simulink model "observerModel_GVS_MS"  (R2023b)
settings: Solver=ode15s  StartTime=0.0  StopTime=duration  MaxStep=0.02  RelTol=0.02  AbsTol=0.02  EnableMultiTasking=on
values from neighbouring files (symbols this model uses):
  beta1 = s(8)    [Observer_Analysis.m]
  beta2 = s(7)    [Observer_Analysis.m]
  delta_t = time(2) - time (1)    [Observer_Analysis.m]
  df = 1    [Observer_Analysis.m]
  f_oto = 2    [Observer_Analysis.m]
  f_scc = 2    [Observer_Analysis.m]
  f_visO = 0.2    [Observer_Analysis.m]
  f_visV = 2    [Observer_Analysis.m]
  f_visX = 2    [Observer_Analysis.m]
  GG0 = [0 0 -hypo]'    [Observer_Analysis.m]
  IrregDepol = tf(num,den)    [Observer_Analysis.m]
  IrregHyperpol = tf(num,den)    [Observer_Analysis.m]
  IrregSCC2Physical = inv(IrregSCCnf)    [Observer_Analysis.m]
  kaa = -3.2*[1 1 1]'    [Observer_Analysis.m]
  Kea = s(1)^(1/2)*[1 1 1]    [Observer_Analysis.m]
  Kef = s(3)^(1/2)*[1 1 1]    [Observer_Analysis.m]
  Kew = s(2)^(1/2)*[1 1 1]    [Observer_Analysis.m]
  Kfast = s(4)    [Observer_Analysis.m]
  kfg = 4*[1 1 1]'    [Observer_Analysis.m]
  kfw = 8*[1 1 1]'    [Observer_Analysis.m]
  kgvg = 5*[1 1 1]'    [Observer_Analysis.m]
  KLeft = 1-KRight    (= 0.5)    [Observer_Analysis.m]
  KReg = s2(2)    [Observer_Analysis.m]
  KRight = 0.5    [Observer_Analysis.m]
  KS = s2(1)*pi/180    [Observer_Analysis.m]
  kwg = 1*[1 1 1]'    [Observer_Analysis.m]
  kwvw = 10*[1 1 1]'    [Observer_Analysis.m]
  kww = 2.28*[1 1 1]'    [Observer_Analysis.m]
  kxdotva = 0.75*[1 1 1]'    [Observer_Analysis.m]
  kxvv = 0.1*[1 1 1]'    [Observer_Analysis.m]
  LeftSide_CurrentMult = s2(4)    [Observer_Analysis.m]
  ms_exp = s(6)    [Observer_Analysis.m]
  oto_a = 60*[1 1 1]'    [Observer_Analysis.m]
  oto_Ka = 1.3*[1 1 1]'    [Observer_Analysis.m]
  Q0 = [cos(E_angle/2) E(1)*sin(E_angle/2) E(2)*sin(E_angle/2) E(3)*sin(E_angle/2)]'    [Observer_Analysis.m]
  RegDepol = tf(num,den)    [Observer_Analysis.m]
  RegHyperpol = tf(num,den)    [Observer_Analysis.m]
  RegSCC2Physical = inv(RegSCCnf)    [Observer_Analysis.m]
  tau_a = tau_a_value*[1 1 1]'    [Observer_Analysis.m]
  tau_scc = tau_scc_value*[1 1 1]'    [Observer_Analysis.m]
  x_leak = 0.6    [Observer_Analysis.m]
  y_leak = 0.6    [Observer_Analysis.m]
  z_leak = 10    [Observer_Analysis.m]
(part 3 of 3)

== system observerModel_GVS_MS/Subsystem5/Subsystem4/Matrix Multiplication ==
  D_Cos : Inport
  a_esr_head : Inport  Port=2
  Demux : Demux  Outputs=3
      settings: DisplayOption=none
  Math Function : Math  Operator=transpose  SignedPower=on
  Mux : Mux  Inputs=3
  Product : Product  Multiplication=Matrix(*)  RndMeth=Zero
  a_est_world : Outport
  wires:
  Product/1 -> Demux/1
  Demux/1 -> Mux/1
  Demux/2 -> Mux/2
  Demux/3 -> Mux/3
  D_Cos/1 -> Math Function/1
  Mux/1 -> a_est_world/1
  a_esr_head/1 -> Product/2
  Math Function/1 -> Product/1

== system observerModel_GVS_MS/To VR (actual)/Limbic to VR Displacement/Transform Axes Translation ==
  head_cord : Inport
  Demux2 : Demux  Outputs=3
  Mux2 : Mux  Inputs=3
  VR_cord : Outport
  wires:
  Demux2/1 -> Mux2/3
  Demux2/2 -> Mux2/1
  Demux2/3 -> Mux2/2
  head_cord/1 -> Demux2/1
  Mux2/1 -> VR_cord/1

== system observerModel_GVS_MS/To VR (est)/Limbic to VR Estimated Displacement/Transform Axes Translation Est ==
  head_cord : Inport
  Demux2 : Demux  Outputs=3
  Mux2 : Mux  Inputs=3
  VR_cord : Outport
  wires:
  Demux2/1 -> Mux2/3
  Demux2/2 -> Mux2/1
  Demux2/3 -> Mux2/2
  head_cord/1 -> Demux2/1
  Mux2/1 -> VR_cord/1

== system observerModel_GVS_MS/Quaternion Rotator/Head to Limbic Angular Velocity Transform/Quaternion Integrator1/delta_q ==
  omega : Inport
  q : Inport  Port=2
  C : Subsystem
  Constant : Constant  Value=delta_t
  K : Subsystem
  Product : Product  RndMeth=Zero
  Product1 : Product  RndMeth=Zero
  Product2 : Product  RndMeth=Zero
  Sum : Sum
  Z : Subsystem
  delta_q : Outport
  wires:
  q/1 -> C/2(q), Z/1(q), Product1/1
  Z/1(z) -> Product/1
  Product/1 -> Product1/2
  Product1/1 -> Sum/2
  C/1(C) -> Sum/1
  Sum/1 -> Product2/2
  Constant/1 -> Product2/1
  omega/1 -> C/1(omega)
  Product2/1 -> delta_q/1
  K/1(K) -> Product/2

== system observerModel_GVS_MS/Quaternion Rotator/Head to Limbic Angular Velocity Transform/Quaternion to Direction Cosine1/A1 ==
  q : Inport
  Demux : Demux
  Gain : Gain  Gain=2
  Product : Product  RndMeth=Zero
  Product1 : Product  RndMeth=Zero
  Sum : Sum  Inputs=+-
  A21 : Outport
  wires:
  q/1 -> Demux/1
  Sum/1 -> Gain/1
  Gain/1 -> A21/1
  Product/1 -> Sum/1
  Product1/1 -> Sum/2
  Demux/2 -> Product/1
  Demux/3 -> Product/2
  Demux/1 -> Product1/1
  Demux/4 -> Product1/2

== system observerModel_GVS_MS/Quaternion Rotator/Head to Limbic Angular Velocity Transform/Quaternion to Direction Cosine1/A11 ==
  q : Inport
  Demux : Demux
  Product{,1..3} (4 alike) : Product  RndMeth=Zero
  Sum : Sum  Inputs=++--
  A11 : Outport
  wires:
  Demux/1 -> Product/1, Product/2
  Demux/2 -> Product1/1, Product1/2
  Demux/3 -> Product2/1, Product2/2
  Demux/4 -> Product3/1, Product3/2
  Product/1 -> Sum/1
  Product1/1 -> Sum/2
  Product2/1 -> Sum/3
  Product3/1 -> Sum/4
  q/1 -> Demux/1
  Sum/1 -> A11/1

== system observerModel_GVS_MS/Quaternion Rotator/Head to Limbic Angular Velocity Transform/Quaternion to Direction Cosine1/A12 ==
  q : Inport
  Demux : Demux
  Gain : Gain  Gain=2
  Product : Product  RndMeth=Zero
  Product1 : Product  RndMeth=Zero
  Sum : Sum
  A12 : Outport
  wires:
  q/1 -> Demux/1
  Sum/1 -> Gain/1
  Gain/1 -> A12/1
  Demux/2 -> Product/1
  Demux/3 -> Product/2
  Demux/1 -> Product1/1
  Demux/4 -> Product1/2
  Product/1 -> Sum/1
  Product1/1 -> Sum/2

== system observerModel_GVS_MS/Quaternion Rotator/Head to Limbic Angular Velocity Transform/Quaternion to Direction Cosine1/A13 ==
  q : Inport
  Demux : Demux
  Gain : Gain  Gain=2
  Product : Product  RndMeth=Zero
  Product1 : Product  RndMeth=Zero
  Sum : Sum  Inputs=+-
  A13 : Outport
  wires:
  q/1 -> Demux/1
  Sum/1 -> Gain/1
  Gain/1 -> A13/1
  Product/1 -> Sum/1
  Product1/1 -> Sum/2
  Demux/2 -> Product/1
  Demux/4 -> Product/2
  Demux/1 -> Product1/1
  Demux/3 -> Product1/2

== system observerModel_GVS_MS/Quaternion Rotator/Head to Limbic Angular Velocity Transform/Quaternion to Direction Cosine1/A22 ==
  q : Inport
  Demux : Demux
  Product{,1..3} (4 alike) : Product  RndMeth=Zero
  Sum : Sum  Inputs=+-+-
  A22 : Outport
  wires:
  Demux/1 -> Product/1, Product/2
  Demux/2 -> Product1/1, Product1/2
  Demux/3 -> Product2/1, Product2/2
  Demux/4 -> Product3/1, Product3/2
  Product/1 -> Sum/1
  Product1/1 -> Sum/2
  Product2/1 -> Sum/3
  Product3/1 -> Sum/4
  q/1 -> Demux/1
  Sum/1 -> A22/1

== system observerModel_GVS_MS/Quaternion Rotator/Head to Limbic Angular Velocity Transform/Quaternion to Direction Cosine1/A23 ==
  q : Inport
  Demux : Demux
  Gain : Gain  Gain=2
  Product : Product  RndMeth=Zero
  Product1 : Product  RndMeth=Zero
  Sum : Sum
  A23 : Outport
  wires:
  q/1 -> Demux/1
  Sum/1 -> Gain/1
  Gain/1 -> A23/1
  Product/1 -> Sum/1
  Product1/1 -> Sum/2
  Demux/3 -> Product1/1
  Demux/4 -> Product1/2
  Demux/1 -> Product/1
  Demux/2 -> Product/2

== system observerModel_GVS_MS/Quaternion Rotator/Head to Limbic Angular Velocity Transform/Quaternion to Direction Cosine1/A31 ==
  q : Inport
  Demux : Demux
  Gain : Gain  Gain=2
  Product : Product  RndMeth=Zero
  Product1 : Product  RndMeth=Zero
  Sum : Sum
  A31 : Outport
  wires:
  q/1 -> Demux/1
  Sum/1 -> Gain/1
  Gain/1 -> A31/1
  Product/1 -> Sum/1
  Product1/1 -> Sum/2
  Demux/1 -> Product/1
  Demux/3 -> Product/2
  Demux/2 -> Product1/1
  Demux/4 -> Product1/2

== system observerModel_GVS_MS/Quaternion Rotator/Head to Limbic Angular Velocity Transform/Quaternion to Direction Cosine1/A32 ==
  q : Inport
  Demux : Demux
  Gain : Gain  Gain=2
  Product : Product  RndMeth=Zero
  Product1 : Product  RndMeth=Zero
  Sum : Sum  Inputs=+-
  A32 : Outport
  wires:
  q/1 -> Demux/1
  Sum/1 -> Gain/1
  Gain/1 -> A32/1
  Product/1 -> Sum/1
  Product1/1 -> Sum/2
  Demux/3 -> Product/1
  Demux/4 -> Product/2
  Demux/1 -> Product1/1
  Demux/2 -> Product1/2

== system observerModel_GVS_MS/Quaternion Rotator/Head to Limbic Angular Velocity Transform/Quaternion to Direction Cosine1/A33 ==
  q : Inport
  Demux : Demux
  Product{,1..3} (4 alike) : Product  RndMeth=Zero
  Sum : Sum  Inputs=+--+
  A33 : Outport
  wires:
  Demux/1 -> Product/1, Product/2
  Demux/2 -> Product1/1, Product1/2
  Demux/3 -> Product2/1, Product2/2
  Demux/4 -> Product3/1, Product3/2
  Product/1 -> Sum/1
  Product1/1 -> Sum/2
  Product2/1 -> Sum/3
  Product3/1 -> Sum/4
  q/1 -> Demux/1
  Sum/1 -> A33/1

== system observerModel_GVS_MS/Quaternion Rotator/Quaternion Integrator/delta_q/C ==
  omega : Inport
  q : Inport  Port=2
  C1 : Subsystem
  C2 : Subsystem
  C3 : Subsystem
  C4 : Subsystem
  Mux : Mux
  C : Outport
  wires:
  omega/1 -> C1/1(omega), C2/1(omega), C3/1(omega), C4/1(omega)
  q/1 -> C4/2(q), C3/2(q), C2/2(q), C1/2(q)
  C1/1(c1) -> Mux/1
  C2/1(c2) -> Mux/2
  C3/1(c3) -> Mux/3
  C4/1(c4) -> Mux/4
  Mux/1 -> C/1

== system observerModel_GVS_MS/Quaternion Rotator/Quaternion Integrator/delta_q/K ==
  Product : Product  RndMeth=Zero
  k : Constant  Value=1/delta_t
  value : Constant  Value=0.9
  K : Outport
  wires:
  k/1 -> Product/1
  Product/1 -> K/1
  value/1 -> Product/2

== system observerModel_GVS_MS/Quaternion Rotator/Quaternion Integrator/delta_q/Z ==
  q : Inport
  Constant : Constant
  Demux : Demux
  Product{,1..3} (4 alike) : Product  RndMeth=Zero
  Sum : Sum  Inputs=++++
  Sum1 : Sum  Inputs=+-
  z : Outport
  wires:
  Demux/1 -> Product/1, Product/2
  Demux/2 -> Product1/1, Product1/2
  Demux/3 -> Product2/1, Product2/2
  Demux/4 -> Product3/1, Product3/2
  q/1 -> Demux/1
  Product/1 -> Sum/1
  Product1/1 -> Sum/2
  Product2/1 -> Sum/3
  Product3/1 -> Sum/4
  Sum/1 -> Sum1/2
  Constant/1 -> Sum1/1
  Sum1/1 -> z/1

== system observerModel_GVS_MS/Quaternion Rotator/Rotation/Azimuthal Integrator/Matrix Multiplication1 ==
  D_Cos : Inport
  omega_rad : Inport  Port=2
  Demux : Demux  Outputs=3
      settings: DisplayOption=none
  Mux : Mux  Inputs=3
  Product : Product  Multiplication=Matrix(*)  RndMeth=Zero
  omega_rad' : Outport
  wires:
  Product/1 -> Demux/1
  Demux/1 -> Mux/1
  Demux/2 -> Mux/2
  Demux/3 -> Mux/3
  D_Cos/1 -> Product/1
  Mux/1 -> omega_rad'/1
  omega_rad/1 -> Product/2

== system observerModel_GVS_MS/Quaternion Rotator2/Head to Limbic Angular Velocity Transform Rotation Matrix/Quaternion Integrator1/delta_q ==
  omega : Inport
  q : Inport  Port=2
  C : Subsystem
  Constant : Constant  Value=delta_t
  K : Subsystem
  Product : Product  RndMeth=Zero
  Product1 : Product  RndMeth=Zero
  Product2 : Product  RndMeth=Zero
  Sum : Sum
  Z : Subsystem
  delta_q : Outport
  wires:
  q/1 -> C/2(q), Z/1(q), Product1/1
  Z/1(z) -> Product/1
  Product/1 -> Product1/2
  Product1/1 -> Sum/2
  C/1(C) -> Sum/1
  Sum/1 -> Product2/2
  Constant/1 -> Product2/1
  omega/1 -> C/1(omega)
  Product2/1 -> delta_q/1
  K/1(K) -> Product/2

== system observerModel_GVS_MS/Quaternion Rotator2/Head to Limbic Angular Velocity Transform Rotation Matrix/Quaternion to Direction Cosine1/A1 ==
  q : Inport
  Demux : Demux
  Gain : Gain  Gain=2
  Product : Product  RndMeth=Zero
  Product1 : Product  RndMeth=Zero
  Sum : Sum  Inputs=+-
  A21 : Outport
  wires:
  q/1 -> Demux/1
  Sum/1 -> Gain/1
  Gain/1 -> A21/1
  Product/1 -> Sum/1
  Product1/1 -> Sum/2
  Demux/2 -> Product/1
  Demux/3 -> Product/2
  Demux/1 -> Product1/1
  Demux/4 -> Product1/2

== system observerModel_GVS_MS/Quaternion Rotator2/Head to Limbic Angular Velocity Transform Rotation Matrix/Quaternion to Direction Cosine1/A11 ==
  q : Inport
  Demux : Demux
  Product{,1..3} (4 alike) : Product  RndMeth=Zero
  Sum : Sum  Inputs=++--
  A11 : Outport
  wires:
  Demux/1 -> Product/1, Product/2
  Demux/2 -> Product1/1, Product1/2
  Demux/3 -> Product2/1, Product2/2
  Demux/4 -> Product3/1, Product3/2
  Product/1 -> Sum/1
  Product1/1 -> Sum/2
  Product2/1 -> Sum/3
  Product3/1 -> Sum/4
  q/1 -> Demux/1
  Sum/1 -> A11/1

== system observerModel_GVS_MS/Quaternion Rotator2/Head to Limbic Angular Velocity Transform Rotation Matrix/Quaternion to Direction Cosine1/A12 ==
  q : Inport
  Demux : Demux
  Gain : Gain  Gain=2
  Product : Product  RndMeth=Zero
  Product1 : Product  RndMeth=Zero
  Sum : Sum
  A12 : Outport
  wires:
  q/1 -> Demux/1
  Sum/1 -> Gain/1
  Gain/1 -> A12/1
  Demux/2 -> Product/1
  Demux/3 -> Product/2
  Demux/1 -> Product1/1
  Demux/4 -> Product1/2
  Product/1 -> Sum/1
  Product1/1 -> Sum/2

== system observerModel_GVS_MS/Quaternion Rotator2/Head to Limbic Angular Velocity Transform Rotation Matrix/Quaternion to Direction Cosine1/A13 ==
  q : Inport
  Demux : Demux
  Gain : Gain  Gain=2
  Product : Product  RndMeth=Zero
  Product1 : Product  RndMeth=Zero
  Sum : Sum  Inputs=+-
  A13 : Outport
  wires:
  q/1 -> Demux/1
  Sum/1 -> Gain/1
  Gain/1 -> A13/1
  Product/1 -> Sum/1
  Product1/1 -> Sum/2
  Demux/2 -> Product/1
  Demux/4 -> Product/2
  Demux/1 -> Product1/1
  Demux/3 -> Product1/2

== system observerModel_GVS_MS/Quaternion Rotator2/Head to Limbic Angular Velocity Transform Rotation Matrix/Quaternion to Direction Cosine1/A22 ==
  q : Inport
  Demux : Demux
  Product{,1..3} (4 alike) : Product  RndMeth=Zero
  Sum : Sum  Inputs=+-+-
  A22 : Outport
  wires:
  Demux/1 -> Product/1, Product/2
  Demux/2 -> Product1/1, Product1/2
  Demux/3 -> Product2/1, Product2/2
  Demux/4 -> Product3/1, Product3/2
  Product/1 -> Sum/1
  Product1/1 -> Sum/2
  Product2/1 -> Sum/3
  Product3/1 -> Sum/4
  q/1 -> Demux/1
  Sum/1 -> A22/1

== system observerModel_GVS_MS/Quaternion Rotator2/Head to Limbic Angular Velocity Transform Rotation Matrix/Quaternion to Direction Cosine1/A23 ==
  q : Inport
  Demux : Demux
  Gain : Gain  Gain=2
  Product : Product  RndMeth=Zero
  Product1 : Product  RndMeth=Zero
  Sum : Sum
  A23 : Outport
  wires:
  q/1 -> Demux/1
  Sum/1 -> Gain/1
  Gain/1 -> A23/1
  Product/1 -> Sum/1
  Product1/1 -> Sum/2
  Demux/3 -> Product1/1
  Demux/4 -> Product1/2
  Demux/1 -> Product/1
  Demux/2 -> Product/2

== system observerModel_GVS_MS/Quaternion Rotator2/Head to Limbic Angular Velocity Transform Rotation Matrix/Quaternion to Direction Cosine1/A31 ==
  q : Inport
  Demux : Demux
  Gain : Gain  Gain=2
  Product : Product  RndMeth=Zero
  Product1 : Product  RndMeth=Zero
  Sum : Sum
  A31 : Outport
  wires:
  q/1 -> Demux/1
  Sum/1 -> Gain/1
  Gain/1 -> A31/1
  Product/1 -> Sum/1
  Product1/1 -> Sum/2
  Demux/1 -> Product/1
  Demux/3 -> Product/2
  Demux/2 -> Product1/1
  Demux/4 -> Product1/2

== system observerModel_GVS_MS/Quaternion Rotator2/Head to Limbic Angular Velocity Transform Rotation Matrix/Quaternion to Direction Cosine1/A32 ==
  q : Inport
  Demux : Demux
  Gain : Gain  Gain=2
  Product : Product  RndMeth=Zero
  Product1 : Product  RndMeth=Zero
  Sum : Sum  Inputs=+-
  A32 : Outport
  wires:
  q/1 -> Demux/1
  Sum/1 -> Gain/1
  Gain/1 -> A32/1
  Product/1 -> Sum/1
  Product1/1 -> Sum/2
  Demux/3 -> Product/1
  Demux/4 -> Product/2
  Demux/1 -> Product1/1
  Demux/2 -> Product1/2

== system observerModel_GVS_MS/Quaternion Rotator2/Head to Limbic Angular Velocity Transform Rotation Matrix/Quaternion to Direction Cosine1/A33 ==
  q : Inport
  Demux : Demux
  Product{,1..3} (4 alike) : Product  RndMeth=Zero
  Sum : Sum  Inputs=+--+
  A33 : Outport
  wires:
  Demux/1 -> Product/1, Product/2
  Demux/2 -> Product1/1, Product1/2
  Demux/3 -> Product2/1, Product2/2
  Demux/4 -> Product3/1, Product3/2
  Product/1 -> Sum/1
  Product1/1 -> Sum/2
  Product2/1 -> Sum/3
  Product3/1 -> Sum/4
  q/1 -> Demux/1
  Sum/1 -> A33/1

== system observerModel_GVS_MS/Quaternion Rotator2/Quaternion Integrator/delta_q/C ==
  omega : Inport
  q : Inport  Port=2
  C1 : Subsystem
  C2 : Subsystem
  C3 : Subsystem
  C4 : Subsystem
  Mux : Mux
  C : Outport
  wires:
  omega/1 -> C1/1(omega), C2/1(omega), C3/1(omega), C4/1(omega)
  q/1 -> C4/2(q), C3/2(q), C2/2(q), C1/2(q)
  C1/1(c1) -> Mux/1
  C2/1(c2) -> Mux/2
  C3/1(c3) -> Mux/3
  C4/1(c4) -> Mux/4
  Mux/1 -> C/1

== system observerModel_GVS_MS/Quaternion Rotator2/Quaternion Integrator/delta_q/K ==
  Product : Product  RndMeth=Zero
  k : Constant  Value=1/delta_t
  value : Constant  Value=0.9
  K : Outport
  wires:
  k/1 -> Product/1
  Product/1 -> K/1
  value/1 -> Product/2

== system observerModel_GVS_MS/Quaternion Rotator2/Quaternion Integrator/delta_q/Z ==
  q : Inport
  Constant : Constant
  Demux : Demux
  Product{,1..3} (4 alike) : Product  RndMeth=Zero
  Sum : Sum  Inputs=++++
  Sum1 : Sum  Inputs=+-
  z : Outport
  wires:
  Demux/1 -> Product/1, Product/2
  Demux/2 -> Product1/1, Product1/2
  Demux/3 -> Product2/1, Product2/2
  Demux/4 -> Product3/1, Product3/2
  q/1 -> Demux/1
  Product/1 -> Sum/1
  Product1/1 -> Sum/2
  Product2/1 -> Sum/3
  Product3/1 -> Sum/4
  Sum/1 -> Sum1/2
  Constant/1 -> Sum1/1
  Sum1/1 -> z/1

== system observerModel_GVS_MS/Quaternion Rotator2/Rotation/Azimuthal Integrator/Matrix Multiplication1 ==
  D_Cos : Inport
  omega_rad : Inport  Port=2
  Demux : Demux  Outputs=3
      settings: DisplayOption=none
  Mux : Mux  Inputs=3
  Product : Product  Multiplication=Matrix(*)  RndMeth=Zero
  omega_rad' : Outport
  wires:
  Product/1 -> Demux/1
  Demux/1 -> Mux/1
  Demux/2 -> Mux/2
  Demux/3 -> Mux/3
  D_Cos/1 -> Product/1
  Mux/1 -> omega_rad'/1
  omega_rad/1 -> Product/2

== system observerModel_GVS_MS/Quaternion Rotator/Head to Limbic Angular Velocity Transform/Quaternion Integrator1/delta_q/C ==
  omega : Inport
  q : Inport  Port=2
  C1 : Subsystem
  C2 : Subsystem
  C3 : Subsystem
  C4 : Subsystem
  Mux : Mux
  C : Outport
  wires:
  omega/1 -> C1/1(omega), C2/1(omega), C3/1(omega), C4/1(omega)
  q/1 -> C4/2(q), C3/2(q), C2/2(q), C1/2(q)
  C1/1(c1) -> Mux/1
  C2/1(c2) -> Mux/2
  C3/1(c3) -> Mux/3
  C4/1(c4) -> Mux/4
  Mux/1 -> C/1

== system observerModel_GVS_MS/Quaternion Rotator/Head to Limbic Angular Velocity Transform/Quaternion Integrator1/delta_q/K ==
  Product : Product  RndMeth=Zero
  k : Constant  Value=1/delta_t
  value : Constant  Value=0.9
  K : Outport
  wires:
  k/1 -> Product/1
  Product/1 -> K/1
  value/1 -> Product/2

== system observerModel_GVS_MS/Quaternion Rotator/Head to Limbic Angular Velocity Transform/Quaternion Integrator1/delta_q/Z ==
  q : Inport
  Constant : Constant
  Demux : Demux
  Product{,1..3} (4 alike) : Product  RndMeth=Zero
  Sum : Sum  Inputs=++++
  Sum1 : Sum  Inputs=+-
  z : Outport
  wires:
  Demux/1 -> Product/1, Product/2
  Demux/2 -> Product1/1, Product1/2
  Demux/3 -> Product2/1, Product2/2
  Demux/4 -> Product3/1, Product3/2
  q/1 -> Demux/1
  Product/1 -> Sum/1
  Product1/1 -> Sum/2
  Product2/1 -> Sum/3
  Product3/1 -> Sum/4
  Sum/1 -> Sum1/2
  Constant/1 -> Sum1/1
  Sum1/1 -> z/1

== system observerModel_GVS_MS/Quaternion Rotator/Quaternion Integrator/delta_q/C/C1 ==
  omega : Inport
  q : Inport  Port=2
  Demux : Demux  Outputs=3
  Demux1 : Demux
  Gain : Gain  Gain=-0.5
  Product : Product  RndMeth=Zero
  Product1 : Product  RndMeth=Zero
  Product2 : Product  RndMeth=Zero
  Sum : Sum  Inputs=+++
  Terminator : Terminator
  c1 : Outport
  wires:
  Demux1/2 -> Product/2
  Demux/1 -> Product/1
  Demux1/3 -> Product1/2
  Demux/2 -> Product1/1
  Demux1/4 -> Product2/2
  Demux/3 -> Product2/1
  Product/1 -> Sum/1
  Product1/1 -> Sum/2
  Product2/1 -> Sum/3
  Sum/1 -> Gain/1
  omega/1 -> Demux/1
  Gain/1 -> c1/1
  q/1 -> Demux1/1
  Demux1/1 -> Terminator/1

== system observerModel_GVS_MS/Quaternion Rotator/Quaternion Integrator/delta_q/C/C2 ==
  omega : Inport
  q : Inport  Port=2
  Demux : Demux  Outputs=3
  Demux1 : Demux
  Gain : Gain  Gain=0.5
  Product : Product  RndMeth=Zero
  Product1 : Product  RndMeth=Zero
  Product2 : Product  RndMeth=Zero
  Sum : Sum  Inputs=++-
  Terminator : Terminator
  c2 : Outport
  wires:
  Product/1 -> Sum/1
  Product1/1 -> Sum/2
  Product2/1 -> Sum/3
  Sum/1 -> Gain/1
  omega/1 -> Demux/1
  Gain/1 -> c2/1
  q/1 -> Demux1/1
  Demux1/1 -> Product/2
  Demux/1 -> Product/1
  Demux1/3 -> Product1/2
  Demux/3 -> Product1/1
  Demux1/4 -> Product2/2
  Demux/2 -> Product2/1
  Demux1/2 -> Terminator/1

== system observerModel_GVS_MS/Quaternion Rotator/Quaternion Integrator/delta_q/C/C3 ==
  omega : Inport
  q : Inport  Port=2
  Demux : Demux  Outputs=3
  Demux1 : Demux
  Gain : Gain  Gain=0.5
  Product : Product  RndMeth=Zero
  Product1 : Product  RndMeth=Zero
  Product2 : Product  RndMeth=Zero
  Sum : Sum  Inputs=++-
  Terminator : Terminator
  c3 : Outport
  wires:
  Product/1 -> Sum/1
  Product1/1 -> Sum/2
  Product2/1 -> Sum/3
  Sum/1 -> Gain/1
  omega/1 -> Demux/1
  Gain/1 -> c3/1
  q/1 -> Demux1/1
  Demux1/1 -> Product/2
  Demux/2 -> Product/1
  Demux1/4 -> Product1/2
  Demux/1 -> Product1/1
  Demux1/2 -> Product2/2
  Demux/3 -> Product2/1
  Demux1/3 -> Terminator/1

== system observerModel_GVS_MS/Quaternion Rotator/Quaternion Integrator/delta_q/C/C4 ==
  omega : Inport
  q : Inport  Port=2
  Demux : Demux  Outputs=3
  Demux1 : Demux
  Gain : Gain  Gain=0.5
  Product : Product  RndMeth=Zero
  Product1 : Product  RndMeth=Zero
  Product2 : Product  RndMeth=Zero
  Sum : Sum  Inputs=++-
  Terminator : Terminator
  c4 : Outport
  wires:
  Product/1 -> Sum/1
  Product1/1 -> Sum/2
  Product2/1 -> Sum/3
  Sum/1 -> Gain/1
  omega/1 -> Demux/1
  Gain/1 -> c4/1
  q/1 -> Demux1/1
  Demux1/1 -> Product/2
  Demux/3 -> Product/1
  Demux1/2 -> Product1/2
  Demux/2 -> Product1/1
  Demux1/3 -> Product2/2
  Demux/1 -> Product2/1
  Demux1/4 -> Terminator/1

== system observerModel_GVS_MS/Quaternion Rotator2/Head to Limbic Angular Velocity Transform Rotation Matrix/Quaternion Integrator1/delta_q/C ==
  omega : Inport
  q : Inport  Port=2
  C1 : Subsystem
  C2 : Subsystem
  C3 : Subsystem
  C4 : Subsystem
  Mux : Mux
  C : Outport
  wires:
  omega/1 -> C1/1(omega), C2/1(omega), C3/1(omega), C4/1(omega)
  q/1 -> C4/2(q), C3/2(q), C2/2(q), C1/2(q)
  C1/1(c1) -> Mux/1
  C2/1(c2) -> Mux/2
  C3/1(c3) -> Mux/3
  C4/1(c4) -> Mux/4
  Mux/1 -> C/1

== system observerModel_GVS_MS/Quaternion Rotator2/Head to Limbic Angular Velocity Transform Rotation Matrix/Quaternion Integrator1/delta_q/K ==
  Product : Product  RndMeth=Zero
  k : Constant  Value=1/delta_t
  value : Constant  Value=0.9
  K : Outport
  wires:
  k/1 -> Product/1
  Product/1 -> K/1
  value/1 -> Product/2

== system observerModel_GVS_MS/Quaternion Rotator2/Head to Limbic Angular Velocity Transform Rotation Matrix/Quaternion Integrator1/delta_q/Z ==
  q : Inport
  Constant : Constant
  Demux : Demux
  Product{,1..3} (4 alike) : Product  RndMeth=Zero
  Sum : Sum  Inputs=++++
  Sum1 : Sum  Inputs=+-
  z : Outport
  wires:
  Demux/1 -> Product/1, Product/2
  Demux/2 -> Product1/1, Product1/2
  Demux/3 -> Product2/1, Product2/2
  Demux/4 -> Product3/1, Product3/2
  q/1 -> Demux/1
  Product/1 -> Sum/1
  Product1/1 -> Sum/2
  Product2/1 -> Sum/3
  Product3/1 -> Sum/4
  Sum/1 -> Sum1/2
  Constant/1 -> Sum1/1
  Sum1/1 -> z/1

== system observerModel_GVS_MS/Quaternion Rotator2/Quaternion Integrator/delta_q/C/C1 ==
  omega : Inport
  q : Inport  Port=2
  Demux : Demux  Outputs=3
  Demux1 : Demux
  Gain : Gain  Gain=-0.5
  Product : Product  RndMeth=Zero
  Product1 : Product  RndMeth=Zero
  Product2 : Product  RndMeth=Zero
  Sum : Sum  Inputs=+++
  Terminator : Terminator
  c1 : Outport
  wires:
  Demux1/2 -> Product/2
  Demux/1 -> Product/1
  Demux1/3 -> Product1/2
  Demux/2 -> Product1/1
  Demux1/4 -> Product2/2
  Demux/3 -> Product2/1
  Product/1 -> Sum/1
  Product1/1 -> Sum/2
  Product2/1 -> Sum/3
  Sum/1 -> Gain/1
  omega/1 -> Demux/1
  Gain/1 -> c1/1
  q/1 -> Demux1/1
  Demux1/1 -> Terminator/1

== system observerModel_GVS_MS/Quaternion Rotator2/Quaternion Integrator/delta_q/C/C2 ==
  omega : Inport
  q : Inport  Port=2
  Demux : Demux  Outputs=3
  Demux1 : Demux
  Gain : Gain  Gain=0.5
  Product : Product  RndMeth=Zero
  Product1 : Product  RndMeth=Zero
  Product2 : Product  RndMeth=Zero
  Sum : Sum  Inputs=++-
  Terminator : Terminator
  c2 : Outport
  wires:
  Product/1 -> Sum/1
  Product1/1 -> Sum/2
  Product2/1 -> Sum/3
  Sum/1 -> Gain/1
  omega/1 -> Demux/1
  Gain/1 -> c2/1
  q/1 -> Demux1/1
  Demux1/1 -> Product/2
  Demux/1 -> Product/1
  Demux1/3 -> Product1/2
  Demux/3 -> Product1/1
  Demux1/4 -> Product2/2
  Demux/2 -> Product2/1
  Demux1/2 -> Terminator/1

== system observerModel_GVS_MS/Quaternion Rotator2/Quaternion Integrator/delta_q/C/C3 ==
  omega : Inport
  q : Inport  Port=2
  Demux : Demux  Outputs=3
  Demux1 : Demux
  Gain : Gain  Gain=0.5
  Product : Product  RndMeth=Zero
  Product1 : Product  RndMeth=Zero
  Product2 : Product  RndMeth=Zero
  Sum : Sum  Inputs=++-
  Terminator : Terminator
  c3 : Outport
  wires:
  Product/1 -> Sum/1
  Product1/1 -> Sum/2
  Product2/1 -> Sum/3
  Sum/1 -> Gain/1
  omega/1 -> Demux/1
  Gain/1 -> c3/1
  q/1 -> Demux1/1
  Demux1/1 -> Product/2
  Demux/2 -> Product/1
  Demux1/4 -> Product1/2
  Demux/1 -> Product1/1
  Demux1/2 -> Product2/2
  Demux/3 -> Product2/1
  Demux1/3 -> Terminator/1

== system observerModel_GVS_MS/Quaternion Rotator2/Quaternion Integrator/delta_q/C/C4 ==
  omega : Inport
  q : Inport  Port=2
  Demux : Demux  Outputs=3
  Demux1 : Demux
  Gain : Gain  Gain=0.5
  Product : Product  RndMeth=Zero
  Product1 : Product  RndMeth=Zero
  Product2 : Product  RndMeth=Zero
  Sum : Sum  Inputs=++-
  Terminator : Terminator
  c4 : Outport
  wires:
  Product/1 -> Sum/1
  Product1/1 -> Sum/2
  Product2/1 -> Sum/3
  Sum/1 -> Gain/1
  omega/1 -> Demux/1
  Gain/1 -> c4/1
  q/1 -> Demux1/1
  Demux1/1 -> Product/2
  Demux/3 -> Product/1
  Demux1/2 -> Product1/2
  Demux/2 -> Product1/1
  Demux1/3 -> Product2/2
  Demux/1 -> Product2/1
  Demux1/4 -> Terminator/1

== system observerModel_GVS_MS/Quaternion Rotator/Head to Limbic Angular Velocity Transform/Quaternion Integrator1/delta_q/C/C1 ==
  omega : Inport
  q : Inport  Port=2
  Demux : Demux  Outputs=3
  Demux1 : Demux
  Gain : Gain  Gain=-0.5
  Product : Product  RndMeth=Zero
  Product1 : Product  RndMeth=Zero
  Product2 : Product  RndMeth=Zero
  Sum : Sum  Inputs=+++
  Terminator : Terminator
  c1 : Outport
  wires:
  Demux1/2 -> Product/2
  Demux/1 -> Product/1
  Demux1/3 -> Product1/2
  Demux/2 -> Product1/1
  Demux1/4 -> Product2/2
  Demux/3 -> Product2/1
  Product/1 -> Sum/1
  Product1/1 -> Sum/2
  Product2/1 -> Sum/3
  Sum/1 -> Gain/1
  omega/1 -> Demux/1
  Gain/1 -> c1/1
  q/1 -> Demux1/1
  Demux1/1 -> Terminator/1

== system observerModel_GVS_MS/Quaternion Rotator/Head to Limbic Angular Velocity Transform/Quaternion Integrator1/delta_q/C/C2 ==
  omega : Inport
  q : Inport  Port=2
  Demux : Demux  Outputs=3
  Demux1 : Demux
  Gain : Gain  Gain=0.5
  Product : Product  RndMeth=Zero
  Product1 : Product  RndMeth=Zero
  Product2 : Product  RndMeth=Zero
  Sum : Sum  Inputs=++-
  Terminator : Terminator
  c2 : Outport
  wires:
  Product/1 -> Sum/1
  Product1/1 -> Sum/2
  Product2/1 -> Sum/3
  Sum/1 -> Gain/1
  omega/1 -> Demux/1
  Gain/1 -> c2/1
  q/1 -> Demux1/1
  Demux1/1 -> Product/2
  Demux/1 -> Product/1
  Demux1/3 -> Product1/2
  Demux/3 -> Product1/1
  Demux1/4 -> Product2/2
  Demux/2 -> Product2/1
  Demux1/2 -> Terminator/1

== system observerModel_GVS_MS/Quaternion Rotator/Head to Limbic Angular Velocity Transform/Quaternion Integrator1/delta_q/C/C3 ==
  omega : Inport
  q : Inport  Port=2
  Demux : Demux  Outputs=3
  Demux1 : Demux
  Gain : Gain  Gain=0.5
  Product : Product  RndMeth=Zero
  Product1 : Product  RndMeth=Zero
  Product2 : Product  RndMeth=Zero
  Sum : Sum  Inputs=++-
  Terminator : Terminator
  c3 : Outport
  wires:
  Product/1 -> Sum/1
  Product1/1 -> Sum/2
  Product2/1 -> Sum/3
  Sum/1 -> Gain/1
  omega/1 -> Demux/1
  Gain/1 -> c3/1
  q/1 -> Demux1/1
  Demux1/1 -> Product/2
  Demux/2 -> Product/1
  Demux1/4 -> Product1/2
  Demux/1 -> Product1/1
  Demux1/2 -> Product2/2
  Demux/3 -> Product2/1
  Demux1/3 -> Terminator/1

== system observerModel_GVS_MS/Quaternion Rotator/Head to Limbic Angular Velocity Transform/Quaternion Integrator1/delta_q/C/C4 ==
  omega : Inport
  q : Inport  Port=2
  Demux : Demux  Outputs=3
  Demux1 : Demux
  Gain : Gain  Gain=0.5
  Product : Product  RndMeth=Zero
  Product1 : Product  RndMeth=Zero
  Product2 : Product  RndMeth=Zero
  Sum : Sum  Inputs=++-
  Terminator : Terminator
  c4 : Outport
  wires:
  Product/1 -> Sum/1
  Product1/1 -> Sum/2
  Product2/1 -> Sum/3
  Sum/1 -> Gain/1
  omega/1 -> Demux/1
  Gain/1 -> c4/1
  q/1 -> Demux1/1
  Demux1/1 -> Product/2
  Demux/3 -> Product/1
  Demux1/2 -> Product1/2
  Demux/2 -> Product1/1
  Demux1/3 -> Product2/2
  Demux/1 -> Product2/1
  Demux1/4 -> Terminator/1

== system observerModel_GVS_MS/Quaternion Rotator2/Head to Limbic Angular Velocity Transform Rotation Matrix/Quaternion Integrator1/delta_q/C/C1 ==
  omega : Inport
  q : Inport  Port=2
  Demux : Demux  Outputs=3
  Demux1 : Demux
  Gain : Gain  Gain=-0.5
  Product : Product  RndMeth=Zero
  Product1 : Product  RndMeth=Zero
  Product2 : Product  RndMeth=Zero
  Sum : Sum  Inputs=+++
  Terminator : Terminator
  c1 : Outport
  wires:
  Demux1/2 -> Product/2
  Demux/1 -> Product/1
  Demux1/3 -> Product1/2
  Demux/2 -> Product1/1
  Demux1/4 -> Product2/2
  Demux/3 -> Product2/1
  Product/1 -> Sum/1
  Product1/1 -> Sum/2
  Product2/1 -> Sum/3
  Sum/1 -> Gain/1
  omega/1 -> Demux/1
  Gain/1 -> c1/1
  q/1 -> Demux1/1
  Demux1/1 -> Terminator/1

== system observerModel_GVS_MS/Quaternion Rotator2/Head to Limbic Angular Velocity Transform Rotation Matrix/Quaternion Integrator1/delta_q/C/C2 ==
  omega : Inport
  q : Inport  Port=2
  Demux : Demux  Outputs=3
  Demux1 : Demux
  Gain : Gain  Gain=0.5
  Product : Product  RndMeth=Zero
  Product1 : Product  RndMeth=Zero
  Product2 : Product  RndMeth=Zero
  Sum : Sum  Inputs=++-
  Terminator : Terminator
  c2 : Outport
  wires:
  Product/1 -> Sum/1
  Product1/1 -> Sum/2
  Product2/1 -> Sum/3
  Sum/1 -> Gain/1
  omega/1 -> Demux/1
  Gain/1 -> c2/1
  q/1 -> Demux1/1
  Demux1/1 -> Product/2
  Demux/1 -> Product/1
  Demux1/3 -> Product1/2
  Demux/3 -> Product1/1
  Demux1/4 -> Product2/2
  Demux/2 -> Product2/1
  Demux1/2 -> Terminator/1

== system observerModel_GVS_MS/Quaternion Rotator2/Head to Limbic Angular Velocity Transform Rotation Matrix/Quaternion Integrator1/delta_q/C/C3 ==
  omega : Inport
  q : Inport  Port=2
  Demux : Demux  Outputs=3
  Demux1 : Demux
  Gain : Gain  Gain=0.5
  Product : Product  RndMeth=Zero
  Product1 : Product  RndMeth=Zero
  Product2 : Product  RndMeth=Zero
  Sum : Sum  Inputs=++-
  Terminator : Terminator
  c3 : Outport
  wires:
  Product/1 -> Sum/1
  Product1/1 -> Sum/2
  Product2/1 -> Sum/3
  Sum/1 -> Gain/1
  omega/1 -> Demux/1
  Gain/1 -> c3/1
  q/1 -> Demux1/1
  Demux1/1 -> Product/2
  Demux/2 -> Product/1
  Demux1/4 -> Product1/2
  Demux/1 -> Product1/1
  Demux1/2 -> Product2/2
  Demux/3 -> Product2/1
  Demux1/3 -> Terminator/1

== system observerModel_GVS_MS/Quaternion Rotator2/Head to Limbic Angular Velocity Transform Rotation Matrix/Quaternion Integrator1/delta_q/C/C4 ==
  omega : Inport
  q : Inport  Port=2
  Demux : Demux  Outputs=3
  Demux1 : Demux
  Gain : Gain  Gain=0.5
  Product : Product  RndMeth=Zero
  Product1 : Product  RndMeth=Zero
  Product2 : Product  RndMeth=Zero
  Sum : Sum  Inputs=++-
  Terminator : Terminator
  c4 : Outport
  wires:
  Product/1 -> Sum/1
  Product1/1 -> Sum/2
  Product2/1 -> Sum/3
  Sum/1 -> Gain/1
  omega/1 -> Demux/1
  Gain/1 -> c4/1
  q/1 -> Demux1/1
  Demux1/1 -> Product/2
  Demux/3 -> Product/1
  Demux1/2 -> Product1/2
  Demux/2 -> Product1/1
  Demux1/3 -> Product2/2
  Demux/1 -> Product2/1
  Demux1/4 -> Terminator/1
